simulink model "gm_sampleModel2003_1_sub"  (R2023a)
settings: Solver=VariableStepAuto  StartTime=0.0  StopTime=10.0  RelTol=1e-3
libraries: simulink x2, hdlsllib x1
settings Model: Creator=user1  LastModifiedBy=user1
settings OptimizationCC: BlockReduction=off  ConditionallyExecuteInputs=off
settings DebuggingCC: InheritedTsInSrcMsg=none

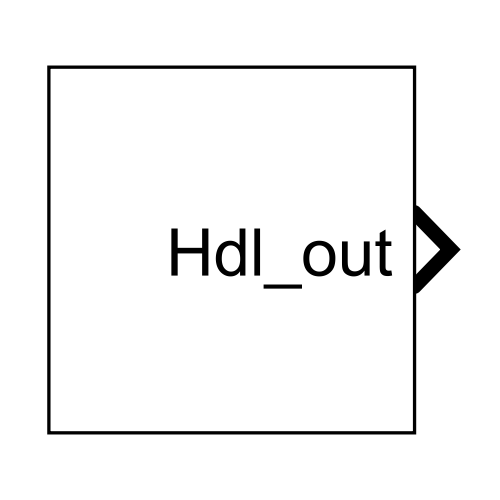
[thumbnail: Simulink's stored preview of the top-level diagram]
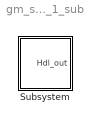
== system gm_sampleModel2003_1_sub ==
  Subsystem : Subsystem

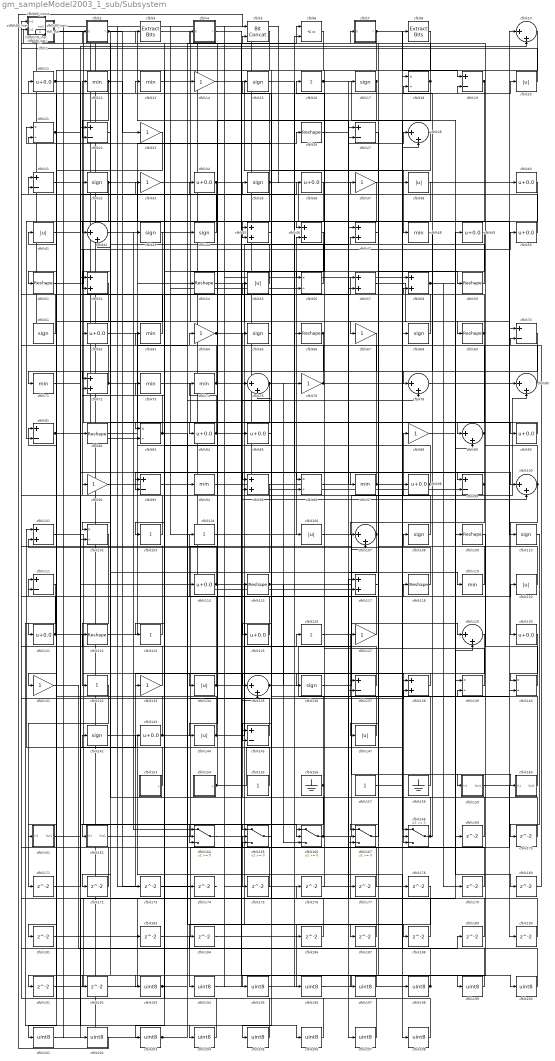
== system gm_sampleModel2003_1_sub/Subsystem ==
  cfblk1 : Subsystem  mask(Compare To Constant){relop=<=, const=double(3), OutDataTypeStr=uint8, ZeroCross=on}
      mask prompts: relop "Simulink:masks:Operator_MP"; const "Simulink:masks:ConstantValue_MP"; OutDataTypeStr "Simulink:masks:OutputDataType_MP"; ZeroCross "Simulink:masks:EnableZerocrossingDetection_MP"
      mask help: Simulink:masks:CompareToConstant_MD
      mask init:
      | OutDataTypeStr = 'uint8';
      | ZeroCross = 'on';
      | blkName = 'sampleModel2003_1_sub/Subsystem/cfblk1';
      | const = double(3);
      | const_str = '3.0';
      | const_val = double(3);
      | relop = '<=';
      | setValue = 'fixdt(0, 8)';
      | str = '<= 3';
      mask TypeOptions relop: == | ~= | < | <= | >= | >
      mask TypeOptions OutDataTypeStr: Simulink:masks:uint8 | Simulink:masks:boolean
      mask Callback ZeroCross: sl('zeroCrossEnable', gcbh);
      mask Display: disp(str)
  cfblk{10,28,42,75,78,80,89,100,107,129,135} (11 alike) : Sum  Inputs=|++  OutDataTypeStr=uint8
  cfblk{45..47,52,57..58,72,95,101,117,138} (11 alike) : Sum  OutDataTypeStr=uint8
  cfblk{18,21,56,83,96,102,139..140} (8 alike) : Product  Inputs=*/  OutDataTypeStr=uint8  RndMeth=Zero  SaturateOnIntegerOverflow=on
  cfblk{16,103..104,123,126,132} (6 alike) : Sum  Inputs=+  OutDataTypeStr=uint8
  cfblk{20,38,41,55,106,120,134,144,147} (9 alike) : Abs  OutDataTypeStr=uint8  SaturateOnIntegerOverflow=off
  cfblk{15,17,32,35,43..44,61,65,68,108,110,136,142} (13 alike) : Signum
  cfblk{26,51,54,59,66,69,82,109,115,118,122} (11 alike) : Reshape
  cfblk{11,34,36,40,49..50,62,84..85,90,98,114,121,125,130,143} (16 alike) : Bias  Bias=0.0  SaturateOnIntegerOverflow=off
  cfblk{19,22,27,31,70,81,93,99,111,137,145} (11 alike) : Sum  Inputs=+-  OutDataTypeStr=uint8
  cfblk113_inst : Subsystem
  cfblk116_inst : Subsystem
  cfblk{12..13,48,63,71,73..74,94,97,119} (10 alike) : MinMax  OutDataTypeStr=uint8
  cfblk124_inst : Subsystem
  cfblk{14,23,33,37,64,67,76,88,92,127,131,133} (12 alike) : Gain  OutDataTypeStr=uint8
  cfblk128_inst : Subsystem
  cfblk141_inst : Subsystem
  cfblk146_inst : Subsystem
  cfblk153 : Subsystem  mask(Counter Limited){uplimit=double(7), tsamp=double(-1)}
      mask prompts: uplimit "Simulink:masks:UpperLimit_MP"; tsamp "Simulink:masks:SampleTime_MP"
      mask help: Simulink:masks:CounterLimited_MD
      mask init:
      | nbits = double(8);
      | tsamp = double(-1);
      | uplimit = double(7);
  cfblk154 : Subsystem  mask(Counter Free-Running){NumBits=double(16), tsamp=double(-1)}
      mask prompts: NumBits "Simulink:masks:NumberOfBits_MP"; tsamp "Simulink:masks:SampleTime_MP"
      mask help: Simulink:masks:CounterFreeRunning_MD
  cfblk155 : Constant  OutDataTypeStr=uint8  SampleTime=-1
  cfblk156 : Ground
  cfblk157 : Constant  OutDataTypeStr=uint8  SampleTime=-1
  cfblk158 : Ground
  cfblk159 : Subsystem
  cfblk160 : Subsystem
  cfblk161 : Subsystem
  cfblk162 : Subsystem
  cfblk{164..168} (5 alike) : Switch  OutDataTypeStr=uint8  SaturateOnIntegerOverflow=off  InputSameDT=off
  cfblk{169..181,183..184,186..192} (22 alike) : Delay  SampleTime=1
  cfblk{193..208} (16 alike) : DataTypeConversion  OutDataTypeStr=uint8  SaturateOnIntegerOverflow=off  RndMeth=Floor
  cfblk2 : Subsystem  mask(Detect Rise Nonnegative){vinit=double(0), InputProcessing=Elements as channels (sample based), OutDataTypeStr=uint8}
      mask prompts: vinit "Simulink:masks:InitialCondition_MP"; InputProcessing "Simulink:masks:InputProcessing_MP"; OutDataTypeStr "Simulink:masks:OutputDataType_MP"
      mask help: Simulink:masks:DetectRiseNonnegative_MD
      mask init:
      | InputProcessing = 'Elements as channels (sample based)';
      | OutDataTypeStr = 'uint8';
      | vinit = double(0);
      mask TypeOptions InputProcessing: Simulink:masks:ColumnsAsChannelsFrameBased | Simulink:masks:ElementsAsChannelsSampleBased
      mask TypeOptions OutDataTypeStr: Simulink:masks:uint8 | Simulink:masks:boolean
      mask Display: fprintf('U >= 0\n&  NOT\nU/z >= 0')
  cfblk24_inst : Subsystem
  cfblk25_inst : Subsystem
  cfblk29_inst : Subsystem
  cfblk3 : simulink/Logic and Bit Operations/Extract Bits  bitsToExtract=Upper half  numBits=8  bitIdxRange=[0 7]  outScalingMode=Preserve fixed-point scaling
      settings: LibrarySourceBlock=|
      | hdlsllib/Logic and Bit
      | Operations/Extract Bits
  cfblk39_inst : Subsystem
  cfblk4 : Subsystem  mask(Detect Fall Nonpositive){vinit=double(0), InputProcessing=Elements as channels (sample based), OutDataTypeStr=uint8}
      mask prompts: vinit "Simulink:masks:InitialCondition_MP"; InputProcessing "Simulink:masks:InputProcessing_MP"; OutDataTypeStr "Simulink:masks:OutputDataType_MP"
      mask help: Simulink:masks:DetectFallNonpositive_MD
      mask init:
      | InputProcessing = 'Elements as channels (sample based)';
      | OutDataTypeStr = 'uint8';
      | vinit = double(0);
      mask TypeOptions InputProcessing: Simulink:masks:ColumnsAsChannelsFrameBased | Simulink:masks:ElementsAsChannelsSampleBased
      mask TypeOptions OutDataTypeStr: Simulink:masks:uint8 | Simulink:masks:boolean
      mask Display: fprintf('U <= 0\n&  NOT\nU/z <= 0')
  cfblk5 : hdlsllib/Logic and Bit Operations/Bit Concat  numInputs=2
  cfblk6 : RelationalOperator  Operator=<=  OutDataTypeStr=boolean  InputSameDT=off
  cfblk60_inst : Subsystem
  cfblk7 : Subsystem  mask(Detect Rise Positive){vinit=double(0), InputProcessing=Elements as channels (sample based), OutDataTypeStr=uint8}
      mask prompts: vinit "Simulink:masks:InitialCondition_MP"; InputProcessing "Simulink:masks:InputProcessing_MP"; OutDataTypeStr "Simulink:masks:OutputDataType_MP"
      mask help: Simulink:masks:DetectRisePositive_MD
      mask init:
      | InputProcessing = 'Elements as channels (sample based)';
      | OutDataTypeStr = 'uint8';
      | vinit = double(0);
      mask TypeOptions InputProcessing: Simulink:masks:ColumnsAsChannelsFrameBased | Simulink:masks:ElementsAsChannelsSampleBased
      mask TypeOptions OutDataTypeStr: Simulink:masks:uint8 | Simulink:masks:boolean
      mask Display: fprintf('U > 0\n&  NOT\nU/z > 0')
  cfblk79_inst : Subsystem
  cfblk8 : simulink/Logic and Bit Operations/Extract Bits  bitsToExtract=Upper half  numBits=8  bitIdxRange=[0 7]  outScalingMode=Preserve fixed-point scaling
      settings: LibrarySourceBlock=|
      | hdlsllib/Logic and Bit
      | Operations/Extract Bits
  cfblk86_inst : Subsystem
  cfblk9_inst : Subsystem
  Hdl_out : Outport  OutDataTypeStr=uint8  SampleTime=1
  wires:
  cfblk1/1(y) -> cfblk89/1, cfblk45/2
  cfblk10/1 -> cfblk75/2
  cfblk100/1 -> cfblk47/2, cfblk130/1, cfblk128_inst/2(in2)
  cfblk101/1 -> cfblk166/2
  cfblk102/1 -> cfblk132/1
  cfblk103/1 -> cfblk12/1
  cfblk104/1 -> cfblk46/2
  cfblk106/1 -> cfblk129/1
  cfblk107/1 -> cfblk25_inst/2(in2), cfblk172/1
  cfblk108/1 -> cfblk35/1
  cfblk109/1 -> cfblk191/1
  cfblk11/1 -> cfblk164/3, cfblk97/1
  cfblk110/1 -> cfblk170/1
  cfblk111/1 -> cfblk204/1
  cfblk113_inst/1(out1) -> cfblk40/1
  cfblk114/1 -> cfblk29_inst/2(in2), cfblk188/1
  cfblk115/1 -> cfblk80/2, cfblk166/3, cfblk159/1(In1)
  cfblk116_inst/1(out1) -> cfblk94/1
  cfblk117/1 -> cfblk7/1(U)
  cfblk118/1 -> cfblk101/2
  cfblk119/1 -> cfblk29_inst/1(in1)
  cfblk12/1 -> cfblk22/2, cfblk23/1
  cfblk120/1 -> cfblk92/1
  cfblk121/1 -> cfblk60_inst/1(in1), cfblk168/3
  cfblk122/1 -> cfblk26/1
  cfblk123/1 -> cfblk41/1
  cfblk124_inst/1(out1) -> cfblk178/1
  cfblk125/1 -> cfblk141_inst/1(in1)
  cfblk126/1 -> cfblk49/1
  cfblk127/1 -> cfblk104/1
  cfblk128_inst/1(out1) -> cfblk43/1
  cfblk129/1 -> cfblk173/1
  cfblk13/1 -> cfblk67/1
  cfblk130/1 -> cfblk140/1
  cfblk131/1 -> cfblk189/1
  cfblk132/1 -> cfblk171/1
  cfblk133/1 -> cfblk39_inst/2(in2)
  cfblk134/1 -> cfblk21/2, cfblk126/1
  cfblk135/1 -> cfblk107/2, cfblk76/1, cfblk139/2
  cfblk136/1 -> cfblk88/1
  cfblk137/1 -> cfblk146_inst/2(in2)
  cfblk138/1 -> cfblk136/1
  cfblk139/1 -> cfblk16/1
  cfblk14/1 -> cfblk48/1
  cfblk140/1 -> cfblk9_inst/1(in1)
  cfblk141_inst/1(out1) -> cfblk82/1
  cfblk142/1 -> cfblk208/1
  cfblk143/1 -> cfblk68/1, cfblk42/2
  cfblk144/1 -> cfblk31/1, cfblk27/1, cfblk122/1
  cfblk145/1 -> cfblk9_inst/2(in2)
  cfblk146_inst/1(out1) -> cfblk202/1
  cfblk147/1 -> cfblk127/1
  cfblk15/1 -> cfblk90/1
  cfblk153/1(y) -> cfblk142/1
  cfblk154/1(y) -> cfblk8/1, cfblk64/1
  cfblk155/1 -> cfblk101/1
  cfblk156/1 -> cfblk21/1, cfblk162/1(In1)
  cfblk157/1 -> cfblk28/2
  cfblk158/1 -> cfblk137/1
  cfblk159/1(Out1) -> cfblk190/1
  cfblk16/1 -> cfblk168/1, cfblk109/1
  cfblk160/1(Out1) -> cfblk32/1
  cfblk161/1(Out1) -> cfblk143/1
  cfblk162/1(Out1) -> cfblk138/2
  cfblk164/1 -> cfblk175/1
  cfblk165/1 -> cfblk195/1
  cfblk166/1 -> cfblk70/1, cfblk2/1(U)
  cfblk167/1 -> cfblk37/1
  cfblk168/1 -> cfblk65/1, cfblk108/1
  cfblk169/1 -> cfblk18/2
  cfblk17/1 -> cfblk84/1, cfblk135/1
  cfblk170/1 -> cfblk95/2
  cfblk171/1 -> cfblk10/2
  cfblk172/1 -> cfblk24_inst/2(in2)
  cfblk173/1 -> cfblk89/2
  cfblk174/1 -> cfblk1/1(u)
  cfblk175/1 -> cfblk39_inst/1(in1)
  cfblk176/1 -> cfblk96/2
  cfblk177/1 -> cfblk75/1
  cfblk178/1 -> cfblk194/1
  cfblk179/1 -> cfblk141_inst/2(in2)
  cfblk18/1 -> cfblk27/2, cfblk145/2, cfblk116_inst/1(in1)
  cfblk180/1 -> cfblk70/2
  cfblk181/1 -> cfblk117/1
  cfblk183/1 -> cfblk140/2
  cfblk184/1 -> cfblk196/1
  cfblk186/1 -> cfblk165/3
  cfblk187/1 -> cfblk81/1
  cfblk188/1 -> cfblk167/2
  cfblk189/1 -> cfblk168/2
  cfblk19/1 -> cfblk81/2, cfblk107/1
  cfblk190/1 -> cfblk116_inst/2(in2)
  cfblk191/1 -> cfblk139/1
  cfblk192/1 -> cfblk165/2
  cfblk193/1 -> cfblk78/2, cfblk57/1, cfblk120/1, cfblk118/1
  cfblk194/1 -> cfblk6/1
  cfblk195/1 -> cfblk6/2
  cfblk196/1 -> cfblk200/1
  cfblk197/1 -> cfblk184/1
  cfblk198/1 -> cfblk86_inst/2(in2), cfblk18/1
  cfblk199/1 -> cfblk79_inst/1(in1)
  cfblk2/1(Y) -> cfblk42/1, cfblk137/2
  cfblk20/1 -> cfblk146_inst/1(in1)
  cfblk200/1 -> cfblk79_inst/2(in2)
  cfblk201/1 -> cfblk176/1
  cfblk202/1 -> cfblk5/1
  cfblk203/1 -> cfblk5/2, Hdl_out/1
  cfblk204/1 -> cfblk124_inst/1(in1)
  cfblk205/1 -> cfblk111/1
  cfblk206/1 -> cfblk111/2
  cfblk207/1 -> cfblk124_inst/2(in2)
  cfblk208/1 -> cfblk3/1
  cfblk21/1 -> cfblk46/1, cfblk206/1, cfblk183/1
  cfblk22/1 -> cfblk102/1
  cfblk23/1 -> cfblk181/1
  cfblk24_inst/1(out1) -> cfblk117/2, cfblk83/2
  cfblk25_inst/1(out1) -> cfblk106/1
  cfblk26/1 -> cfblk119/1
  cfblk27/1 -> cfblk187/1
  cfblk28/1 -> cfblk45/1
  cfblk29_inst/1(out1) -> cfblk58/1
  cfblk3/1 -> cfblk207/1
  cfblk31/1 -> cfblk114/1
  cfblk32/1 -> cfblk177/1, cfblk102/2
  cfblk33/1 -> cfblk59/1
  cfblk34/1 -> cfblk203/1, cfblk138/1
  cfblk35/1 -> cfblk80/1, cfblk144/1, cfblk113_inst/1(in1)
  cfblk36/1 -> cfblk52/2
  cfblk37/1 -> cfblk51/1
  cfblk38/1 -> cfblk134/1
  cfblk39_inst/1(out1) -> cfblk44/1, cfblk56/2
  cfblk4/1(Y) -> cfblk199/1
  cfblk40/1 -> cfblk161/1(In1)
  cfblk41/1 -> cfblk69/1
  cfblk42/1 -> cfblk164/1
  cfblk43/1 -> cfblk131/1
  cfblk44/1 -> cfblk24_inst/1(in1)
  cfblk45/1 -> cfblk165/1
  cfblk46/1 -> cfblk123/1
  cfblk47/1 -> cfblk147/1
  cfblk48/1 -> cfblk78/1
  cfblk49/1 -> cfblk197/1
  cfblk5/1 -> cfblk201/1
  cfblk50/1 -> cfblk11/1
  cfblk51/1 -> cfblk17/1
  cfblk52/1 -> cfblk121/1
  cfblk54/1 -> cfblk110/1
  cfblk55/1 -> cfblk25_inst/1(in1)
  cfblk56/1 -> cfblk13/1
  cfblk57/1 -> cfblk169/1
  cfblk58/1 -> cfblk180/1, cfblk179/1
  cfblk59/1 -> cfblk4/1(U)
  cfblk6/1 -> cfblk193/1
  cfblk60_inst/1(out1) -> cfblk174/1
  cfblk61/1 -> cfblk86_inst/1(in1)
  cfblk62/1 -> cfblk115/1
  cfblk63/1 -> cfblk52/1
  cfblk64/1 -> cfblk20/1, cfblk100/1
  cfblk65/1 -> cfblk15/1
  cfblk66/1 -> cfblk95/1, cfblk93/2
  cfblk67/1 -> cfblk72/1
  cfblk68/1 -> cfblk60_inst/2(in2)
  cfblk69/1 -> cfblk58/2, cfblk205/1, cfblk103/1
  cfblk7/1(Y) -> cfblk19/1, cfblk56/1
  cfblk70/1 -> cfblk71/1
  cfblk71/1 -> cfblk50/1
  cfblk72/1 -> cfblk54/1, cfblk22/1
  cfblk73/1 -> cfblk129/2
  cfblk74/1 -> cfblk62/1, cfblk135/2
  cfblk75/1 -> cfblk99/1, cfblk192/1
  cfblk76/1 -> cfblk57/2, cfblk31/2, cfblk19/2, cfblk63/1
  cfblk78/1 -> cfblk10/1
  cfblk79_inst/1(out1) -> cfblk198/1
  cfblk8/1 -> cfblk145/1
  cfblk80/1 -> cfblk128_inst/1(in1)
  cfblk81/1 -> cfblk55/1, cfblk36/1
  cfblk82/1 -> cfblk14/1
  cfblk83/1 -> cfblk72/2, cfblk166/1, cfblk186/1
  cfblk84/1 -> cfblk66/1, cfblk74/1
  cfblk85/1 -> cfblk125/1
  cfblk86_inst/1(out1) -> cfblk98/1
  cfblk88/1 -> cfblk160/1(In1)
  cfblk89/1 -> cfblk167/3, cfblk33/1
  cfblk9_inst/1(out1) -> cfblk99/2, cfblk61/1
  cfblk90/1 -> cfblk83/1
  cfblk92/1 -> cfblk85/1
  cfblk93/1 -> cfblk164/2
  cfblk94/1 -> cfblk100/2
  cfblk95/1 -> cfblk133/1
  cfblk96/1 -> cfblk28/1
  cfblk97/1 -> cfblk38/1, cfblk34/1, cfblk113_inst/2(in2)
  cfblk98/1 -> cfblk47/1, cfblk96/1, cfblk73/1
  cfblk99/1 -> cfblk93/1, cfblk167/1

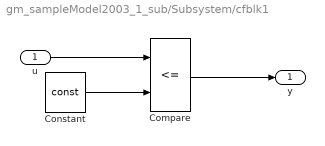
== system gm_sampleModel2003_1_sub/Subsystem/cfblk1 ==
  u : Inport  OutDataTypeStr=uint8  SampleTime=1
  Compare : RelationalOperator  Operator=<=  OutDataTypeStr=fixdt(0, 8)
  Constant : Constant  DisableCoverage=on  Value=const  OutDataTypeStr=Inherit: Inherit via back propagation  SampleTime=-1
  y : Outport  SampleTime=1
  wires:
  u/1 -> Compare/1
  Compare/1 -> y/1
  Constant/1 -> Compare/2

== system gm_sampleModel2003_1_sub/Subsystem/cfblk113_inst ==
  in1 : Inport  OutDataTypeStr=uint8  SampleTime=1
  in2 : Inport  Port=2  OutDataTypeStr=uint8  SampleTime=1
  mul_cfblk113_dotp_mulcomp : Product  Inputs=**  OutDataTypeStr=uint8  SampleTime=1
  out1 : Outport  OutDataTypeStr=uint8  SampleTime=1
  wires:
  in1/1 -> mul_cfblk113_dotp_mulcomp/1
  in2/1 -> mul_cfblk113_dotp_mulcomp/2
  mul_cfblk113_dotp_mulcomp/1 -> out1/1

== system gm_sampleModel2003_1_sub/Subsystem/cfblk116_inst ==
  in1 : Inport  OutDataTypeStr=uint8  SampleTime=1
  in2 : Inport  Port=2  OutDataTypeStr=uint8  SampleTime=1
  mul_cfblk116_dotp_mulcomp : Product  Inputs=**  OutDataTypeStr=uint8  SampleTime=1
  out1 : Outport  OutDataTypeStr=uint8  SampleTime=1
  wires:
  in1/1 -> mul_cfblk116_dotp_mulcomp/1
  in2/1 -> mul_cfblk116_dotp_mulcomp/2
  mul_cfblk116_dotp_mulcomp/1 -> out1/1

== system gm_sampleModel2003_1_sub/Subsystem/cfblk124_inst ==
  in1 : Inport  OutDataTypeStr=uint8  SampleTime=1
  in2 : Inport  Port=2  OutDataTypeStr=uint8  SampleTime=1
  mul_cfblk124_dotp_mulcomp : Product  Inputs=**  OutDataTypeStr=uint8  SampleTime=1
  out1 : Outport  OutDataTypeStr=uint8  SampleTime=1
  wires:
  in1/1 -> mul_cfblk124_dotp_mulcomp/1
  in2/1 -> mul_cfblk124_dotp_mulcomp/2
  mul_cfblk124_dotp_mulcomp/1 -> out1/1

== system gm_sampleModel2003_1_sub/Subsystem/cfblk128_inst ==
  in1 : Inport  OutDataTypeStr=uint8  SampleTime=1
  in2 : Inport  Port=2  OutDataTypeStr=uint8  SampleTime=1
  mul_cfblk128_dotp_mulcomp : Product  Inputs=**  OutDataTypeStr=uint8  SampleTime=1
  out1 : Outport  OutDataTypeStr=uint8  SampleTime=1
  wires:
  in1/1 -> mul_cfblk128_dotp_mulcomp/1
  in2/1 -> mul_cfblk128_dotp_mulcomp/2
  mul_cfblk128_dotp_mulcomp/1 -> out1/1

== system gm_sampleModel2003_1_sub/Subsystem/cfblk141_inst ==
  in1 : Inport  OutDataTypeStr=uint8  SampleTime=1
  in2 : Inport  Port=2  OutDataTypeStr=uint8  SampleTime=1
  mul_cfblk141_dotp_mulcomp : Product  Inputs=**  OutDataTypeStr=uint8  SampleTime=1
  out1 : Outport  OutDataTypeStr=uint8  SampleTime=1
  wires:
  in1/1 -> mul_cfblk141_dotp_mulcomp/1
  in2/1 -> mul_cfblk141_dotp_mulcomp/2
  mul_cfblk141_dotp_mulcomp/1 -> out1/1

== system gm_sampleModel2003_1_sub/Subsystem/cfblk146_inst ==
  in1 : Inport  OutDataTypeStr=uint8  SampleTime=1
  in2 : Inport  Port=2  OutDataTypeStr=uint8  SampleTime=1
  mul_cfblk146_dotp_mulcomp : Product  Inputs=**  OutDataTypeStr=uint8  SampleTime=1
  out1 : Outport  OutDataTypeStr=uint8  SampleTime=1
  wires:
  in1/1 -> mul_cfblk146_dotp_mulcomp/1
  in2/1 -> mul_cfblk146_dotp_mulcomp/2
  mul_cfblk146_dotp_mulcomp/1 -> out1/1

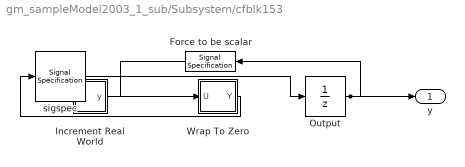
== system gm_sampleModel2003_1_sub/Subsystem/cfblk153 ==
  Force to be scalar : SignalSpecification  DisableCoverage=on  Dimensions=1
  Increment Real World : Subsystem  mask(Real World Value Increment){}
      mask help: Simulink:masks:RealWorldValueIncrement_MD
      mask Display: disp('V++')
  Output : UnitDelay  InitialCondition=0.0  SampleTime=tsamp  HasFrameUpgradeWarning=on
  Wrap To Zero : Subsystem  mask(Wrap To Zero){Threshold=double(7)}
      mask prompts: Threshold "Simulink:masks:Threshold_MP"
      mask help: Simulink:masks:WrapToZero_MD
  sigspec : SignalSpecification  OutDataTypeStr=uint8  Dimensions=1
  y : Outport  SampleTime=1
  wires:
  Force to be scalar/1 -> Increment Real World/1(u)
  Increment Real World/1(y) -> Wrap To Zero/1(U)
  Output/1 -> Force to be scalar/1, y/1
  Wrap To Zero/1(Y) -> sigspec/1
  sigspec/1 -> Output/1

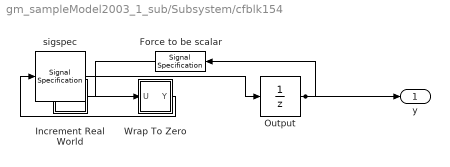
== system gm_sampleModel2003_1_sub/Subsystem/cfblk154 ==
  Force to be scalar : SignalSpecification  DisableCoverage=on  Dimensions=1
  Increment Real World : Subsystem  mask(Real World Value Increment){}
      mask help: Simulink:masks:RealWorldValueIncrement_MD
      mask Display: disp('V++')
  Output : UnitDelay  InitialCondition=0.0  SampleTime=tsamp  HasFrameUpgradeWarning=on
  Wrap To Zero : Subsystem  mask(Wrap To Zero){Threshold=double(65535)}
      mask prompts: Threshold "Simulink:masks:Threshold_MP"
      mask help: Simulink:masks:WrapToZero_MD
  sigspec : SignalSpecification  OutDataTypeStr=uint16  Dimensions=1
  y : Outport  SampleTime=1
  wires:
  Force to be scalar/1 -> Increment Real World/1(u)
  Increment Real World/1(y) -> Wrap To Zero/1(U)
  Output/1 -> Force to be scalar/1, y/1
  Wrap To Zero/1(Y) -> sigspec/1
  sigspec/1 -> Output/1

== system gm_sampleModel2003_1_sub/Subsystem/cfblk159 ==
  In1 : Inport  OutDataTypeStr=uint8  PortDimensions=1  SampleTime=1
  Out1 : Outport  SampleTime=1
  wires:
  In1/1 -> Out1/1

== system gm_sampleModel2003_1_sub/Subsystem/cfblk160 ==
  In1 : Inport  OutDataTypeStr=uint8  PortDimensions=1  SampleTime=1
  Out1 : Outport  SampleTime=1
  wires:
  In1/1 -> Out1/1

== system gm_sampleModel2003_1_sub/Subsystem/cfblk161 ==
  In1 : Inport  OutDataTypeStr=uint8  PortDimensions=1  SampleTime=1
  Out1 : Outport  SampleTime=1
  wires:
  In1/1 -> Out1/1

== system gm_sampleModel2003_1_sub/Subsystem/cfblk162 ==
  In1 : Inport  OutDataTypeStr=uint8  PortDimensions=1  SampleTime=1
  Out1 : Outport  SampleTime=1
  wires:
  In1/1 -> Out1/1

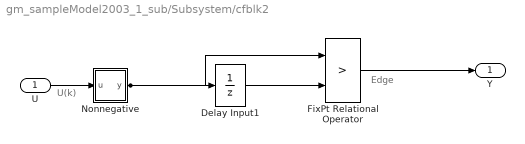
== system gm_sampleModel2003_1_sub/Subsystem/cfblk2 ==
  note: U(k)
  note: Edge
  U : Inport  OutDataTypeStr=uint8  SampleTime=1
  Delay Input1 : UnitDelay  Description=Store in Global RAM  DisableCoverage=on  InitialCondition=vinit  SampleTime=-1  HasFrameUpgradeWarning=on
  FixPt Relational Operator : RelationalOperator  Operator=>  OutDataTypeStr=fixdt(0, 8)  ZeroCross=off  InputSameDT=off
  Nonnegative : Subsystem  mask(Compare To Zero){relop=>=, OutDataTypeStr=boolean, ZeroCross=off}
      mask prompts: relop "Simulink:masks:Operator_MP"; OutDataTypeStr "Simulink:masks:OutputDataType_MP"; ZeroCross "Simulink:masks:EnableZerocrossingDetection_MP"
      mask help: Simulink:masks:CompareToZero_MD
      mask init:
      | OutDataTypeStr = 'boolean';
      | ZeroCross = 'off';
      | blkName = 'sampleModel2003_1_sub/Subsystem/cfblk2/Nonnegative';
      | relop = '>=';
      | setValue = 'boolean';
      mask TypeOptions relop: == | ~= | < | <= | >= | >
      mask TypeOptions OutDataTypeStr: Simulink:masks:uint8 | Simulink:masks:boolean
      mask Callback ZeroCross: sl('zeroCrossEnable', gcbh);
      mask Display: disp([relop,' 0'])
  Y : Outport  SampleTime=1
  wires:
  U/1 -> Nonnegative/1(u)
  Delay Input1/1 -> FixPt Relational Operator/2
  FixPt Relational Operator/1 -> Y/1
  Nonnegative/1(y) -> FixPt Relational Operator/1, Delay Input1/1

== system gm_sampleModel2003_1_sub/Subsystem/cfblk24_inst ==
  in1 : Inport  OutDataTypeStr=uint8  SampleTime=1
  in2 : Inport  Port=2  OutDataTypeStr=uint8  SampleTime=1
  mul_cfblk24_dotp_mulcomp : Product  Inputs=**  OutDataTypeStr=uint8  SampleTime=1
  out1 : Outport  OutDataTypeStr=uint8  SampleTime=1
  wires:
  in1/1 -> mul_cfblk24_dotp_mulcomp/1
  in2/1 -> mul_cfblk24_dotp_mulcomp/2
  mul_cfblk24_dotp_mulcomp/1 -> out1/1

== system gm_sampleModel2003_1_sub/Subsystem/cfblk25_inst ==
  in1 : Inport  OutDataTypeStr=uint8  SampleTime=1
  in2 : Inport  Port=2  OutDataTypeStr=uint8  SampleTime=1
  mul_cfblk25_dotp_mulcomp : Product  Inputs=**  OutDataTypeStr=uint8  SampleTime=1
  out1 : Outport  OutDataTypeStr=uint8  SampleTime=1
  wires:
  in1/1 -> mul_cfblk25_dotp_mulcomp/1
  in2/1 -> mul_cfblk25_dotp_mulcomp/2
  mul_cfblk25_dotp_mulcomp/1 -> out1/1

== system gm_sampleModel2003_1_sub/Subsystem/cfblk29_inst ==
  in1 : Inport  OutDataTypeStr=uint8  SampleTime=1
  in2 : Inport  Port=2  OutDataTypeStr=uint8  SampleTime=1
  mul_cfblk29_dotp_mulcomp : Product  Inputs=**  OutDataTypeStr=uint8  SampleTime=1
  out1 : Outport  OutDataTypeStr=uint8  SampleTime=1
  wires:
  in1/1 -> mul_cfblk29_dotp_mulcomp/1
  in2/1 -> mul_cfblk29_dotp_mulcomp/2
  mul_cfblk29_dotp_mulcomp/1 -> out1/1

== system gm_sampleModel2003_1_sub/Subsystem/cfblk39_inst ==
  in1 : Inport  OutDataTypeStr=uint8  SampleTime=1
  in2 : Inport  Port=2  OutDataTypeStr=uint8  SampleTime=1
  mul_cfblk39_dotp_mulcomp : Product  Inputs=**  OutDataTypeStr=uint8  SampleTime=1
  out1 : Outport  OutDataTypeStr=uint8  SampleTime=1
  wires:
  in1/1 -> mul_cfblk39_dotp_mulcomp/1
  in2/1 -> mul_cfblk39_dotp_mulcomp/2
  mul_cfblk39_dotp_mulcomp/1 -> out1/1

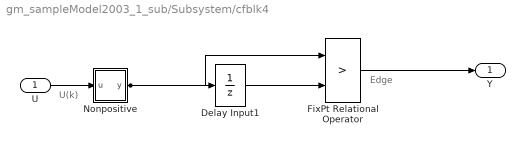
== system gm_sampleModel2003_1_sub/Subsystem/cfblk4 ==
  note: U(k)
  note: Edge
  U : Inport  OutDataTypeStr=uint8  SampleTime=1
  Delay Input1 : UnitDelay  Description=Store in Global RAM  DisableCoverage=on  InitialCondition=vinit  SampleTime=-1  HasFrameUpgradeWarning=on
  FixPt Relational Operator : RelationalOperator  Operator=>  OutDataTypeStr=fixdt(0, 8)  ZeroCross=off  InputSameDT=off
  Nonpositive : Subsystem  mask(Compare To Zero){relop=<=, OutDataTypeStr=boolean, ZeroCross=off}
      mask prompts: relop "Simulink:masks:Operator_MP"; OutDataTypeStr "Simulink:masks:OutputDataType_MP"; ZeroCross "Simulink:masks:EnableZerocrossingDetection_MP"
      mask help: Simulink:masks:CompareToZero_MD
      mask init:
      | OutDataTypeStr = 'boolean';
      | ZeroCross = 'off';
      | blkName = 'sampleModel2003_1_sub/Subsystem/cfblk4/Nonpositive';
      | relop = '<=';
      | setValue = 'boolean';
      mask TypeOptions relop: == | ~= | < | <= | >= | >
      mask TypeOptions OutDataTypeStr: Simulink:masks:uint8 | Simulink:masks:boolean
      mask Callback ZeroCross: sl('zeroCrossEnable', gcbh);
      mask Display: disp([relop,' 0'])
  Y : Outport  SampleTime=1
  wires:
  U/1 -> Nonpositive/1(u)
  Delay Input1/1 -> FixPt Relational Operator/2
  FixPt Relational Operator/1 -> Y/1
  Nonpositive/1(y) -> FixPt Relational Operator/1, Delay Input1/1

== system gm_sampleModel2003_1_sub/Subsystem/cfblk60_inst ==
  in1 : Inport  OutDataTypeStr=uint8  SampleTime=1
  in2 : Inport  Port=2  OutDataTypeStr=uint8  SampleTime=1
  mul_cfblk60_dotp_mulcomp : Product  Inputs=**  OutDataTypeStr=uint8  SampleTime=1
  out1 : Outport  OutDataTypeStr=uint8  SampleTime=1
  wires:
  in1/1 -> mul_cfblk60_dotp_mulcomp/1
  in2/1 -> mul_cfblk60_dotp_mulcomp/2
  mul_cfblk60_dotp_mulcomp/1 -> out1/1

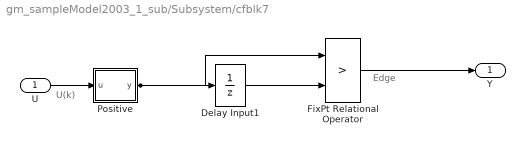
== system gm_sampleModel2003_1_sub/Subsystem/cfblk7 ==
  note: U(k)
  note: Edge
  U : Inport  OutDataTypeStr=uint8  SampleTime=1
  Delay Input1 : UnitDelay  Description=Store in Global RAM  DisableCoverage=on  InitialCondition=vinit  SampleTime=-1  HasFrameUpgradeWarning=on
  FixPt Relational Operator : RelationalOperator  Operator=>  OutDataTypeStr=fixdt(0, 8)  ZeroCross=off  InputSameDT=off
  Positive : Subsystem  mask(Compare To Zero){relop=>, OutDataTypeStr=boolean, ZeroCross=off}
      mask prompts: relop "Simulink:masks:Operator_MP"; OutDataTypeStr "Simulink:masks:OutputDataType_MP"; ZeroCross "Simulink:masks:EnableZerocrossingDetection_MP"
      mask help: Simulink:masks:CompareToZero_MD
      mask init:
      | OutDataTypeStr = 'boolean';
      | ZeroCross = 'off';
      | blkName = 'sampleModel2003_1_sub/Subsystem/cfblk7/Positive';
      | relop = '>';
      | setValue = 'boolean';
      mask TypeOptions relop: == | ~= | < | <= | >= | >
      mask TypeOptions OutDataTypeStr: Simulink:masks:uint8 | Simulink:masks:boolean
      mask Callback ZeroCross: sl('zeroCrossEnable', gcbh);
      mask Display: disp([relop,' 0'])
  Y : Outport  SampleTime=1
  wires:
  U/1 -> Positive/1(u)
  Delay Input1/1 -> FixPt Relational Operator/2
  FixPt Relational Operator/1 -> Y/1
  Positive/1(y) -> FixPt Relational Operator/1, Delay Input1/1

== system gm_sampleModel2003_1_sub/Subsystem/cfblk79_inst ==
  in1 : Inport  OutDataTypeStr=uint8  SampleTime=1
  in2 : Inport  Port=2  OutDataTypeStr=uint8  SampleTime=1
  mul_cfblk79_dotp_mulcomp : Product  Inputs=**  OutDataTypeStr=uint8  SampleTime=1
  out1 : Outport  OutDataTypeStr=uint8  SampleTime=1
  wires:
  in1/1 -> mul_cfblk79_dotp_mulcomp/1
  in2/1 -> mul_cfblk79_dotp_mulcomp/2
  mul_cfblk79_dotp_mulcomp/1 -> out1/1

== system gm_sampleModel2003_1_sub/Subsystem/cfblk86_inst ==
  in1 : Inport  OutDataTypeStr=uint8  SampleTime=1
  in2 : Inport  Port=2  OutDataTypeStr=uint8  SampleTime=1
  mul_cfblk86_dotp_mulcomp : Product  Inputs=**  OutDataTypeStr=uint8  SampleTime=1
  out1 : Outport  OutDataTypeStr=uint8  SampleTime=1
  wires:
  in1/1 -> mul_cfblk86_dotp_mulcomp/1
  in2/1 -> mul_cfblk86_dotp_mulcomp/2
  mul_cfblk86_dotp_mulcomp/1 -> out1/1

== system gm_sampleModel2003_1_sub/Subsystem/cfblk9_inst ==
  in1 : Inport  OutDataTypeStr=uint8  SampleTime=1
  in2 : Inport  Port=2  OutDataTypeStr=uint8  SampleTime=1
  mul_cfblk9_dotp_mulcomp : Product  Inputs=**  OutDataTypeStr=uint8  SampleTime=1
  out1 : Outport  OutDataTypeStr=uint8  SampleTime=1
  wires:
  in1/1 -> mul_cfblk9_dotp_mulcomp/1
  in2/1 -> mul_cfblk9_dotp_mulcomp/2
  mul_cfblk9_dotp_mulcomp/1 -> out1/1

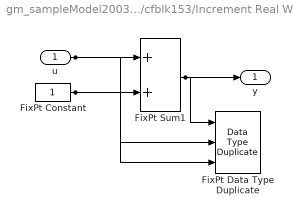
== system gm_sampleModel2003_1_sub/Subsystem/cfblk153/Increment Real World ==
  u : Inport  OutDataTypeStr=uint8  SampleTime=1
  FixPt Constant : Constant  DisableCoverage=on  OutDataTypeStr=Inherit: Inherit via back propagation  SampleTime=-1
  FixPt Data Type Duplicate : DataTypeDuplicate  DisableCoverage=on  NumInputPorts=3
  FixPt Sum1 : Sum  InputSameDT=on  OutDataTypeStr=Inherit: Inherit via back propagation  LockScale=on
  y : Outport  SampleTime=1
  wires:
  u/1 -> FixPt Sum1/1, FixPt Data Type Duplicate/2
  FixPt Constant/1 -> FixPt Sum1/2, FixPt Data Type Duplicate/3
  FixPt Sum1/1 -> FixPt Data Type Duplicate/1, y/1

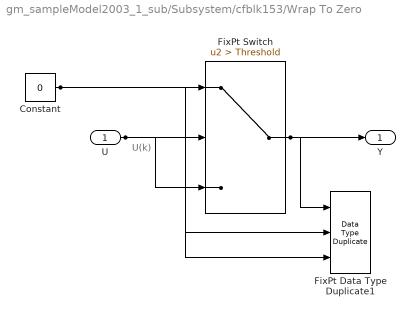
== system gm_sampleModel2003_1_sub/Subsystem/cfblk153/Wrap To Zero ==
  note: U(k)
  U : Inport  OutDataTypeStr=uint8  SampleTime=1
  Constant : Constant  DisableCoverage=on  Value=0  OutDataTypeStr=Inherit: Inherit via back propagation  SampleTime=-1
  FixPt Data Type Duplicate1 : DataTypeDuplicate  DisableCoverage=on  NumInputPorts=3
  FixPt Switch : Switch  Criteria=u2 > Threshold  Threshold=Threshold  OutDataTypeStr=Inherit: Inherit via back propagation  ZeroCross=off  SaturateOnIntegerOverflow=off  InputSameDT=off
  Y : Outport  SampleTime=1
  wires:
  U/1 -> FixPt Switch/3, FixPt Switch/2, FixPt Data Type Duplicate1/2
  Constant/1 -> FixPt Switch/1, FixPt Data Type Duplicate1/3
  FixPt Switch/1 -> FixPt Data Type Duplicate1/1, Y/1

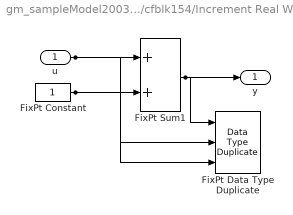
== system gm_sampleModel2003_1_sub/Subsystem/cfblk154/Increment Real World ==
  u : Inport  OutDataTypeStr=uint16  SampleTime=1
  FixPt Constant : Constant  DisableCoverage=on  OutDataTypeStr=Inherit: Inherit via back propagation  SampleTime=-1
  FixPt Data Type Duplicate : DataTypeDuplicate  DisableCoverage=on  NumInputPorts=3
  FixPt Sum1 : Sum  InputSameDT=on  OutDataTypeStr=Inherit: Inherit via back propagation  LockScale=on
  y : Outport  SampleTime=1
  wires:
  u/1 -> FixPt Sum1/1, FixPt Data Type Duplicate/2
  FixPt Constant/1 -> FixPt Sum1/2, FixPt Data Type Duplicate/3
  FixPt Sum1/1 -> FixPt Data Type Duplicate/1, y/1

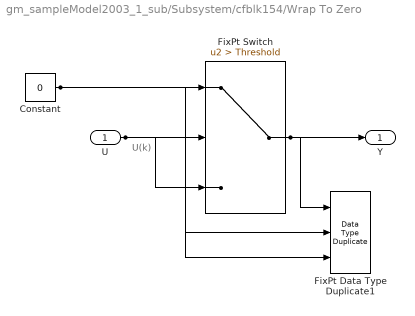
== system gm_sampleModel2003_1_sub/Subsystem/cfblk154/Wrap To Zero ==
  note: U(k)
  U : Inport  OutDataTypeStr=uint16  SampleTime=1
  Constant : Constant  DisableCoverage=on  Value=0  OutDataTypeStr=Inherit: Inherit via back propagation  SampleTime=-1
  FixPt Data Type Duplicate1 : DataTypeDuplicate  DisableCoverage=on  NumInputPorts=3
  FixPt Switch : Switch  Criteria=u2 > Threshold  Threshold=Threshold  OutDataTypeStr=Inherit: Inherit via back propagation  ZeroCross=off  SaturateOnIntegerOverflow=off  InputSameDT=off
  Y : Outport  SampleTime=1
  wires:
  U/1 -> FixPt Switch/3, FixPt Switch/2, FixPt Data Type Duplicate1/2
  Constant/1 -> FixPt Switch/1, FixPt Data Type Duplicate1/3
  FixPt Switch/1 -> FixPt Data Type Duplicate1/1, Y/1

== system gm_sampleModel2003_1_sub/Subsystem/cfblk2/Nonnegative ==
  u : Inport  OutDataTypeStr=uint8  SampleTime=1
  Compare : RelationalOperator  OutDataTypeStr=boolean  ZeroCross=off
  Constant : Constant  DisableCoverage=on  Value=0  OutDataTypeStr=Inherit: Inherit via back propagation  SampleTime=-1  PreserveConstantTs=on
  y : Outport  SampleTime=1
  wires:
  u/1 -> Compare/1
  Compare/1 -> y/1
  Constant/1 -> Compare/2

== system gm_sampleModel2003_1_sub/Subsystem/cfblk4/Nonpositive ==
  u : Inport  OutDataTypeStr=uint8  SampleTime=1
  Compare : RelationalOperator  Operator=<=  OutDataTypeStr=boolean  ZeroCross=off
  Constant : Constant  DisableCoverage=on  Value=0  OutDataTypeStr=Inherit: Inherit via back propagation  SampleTime=-1  PreserveConstantTs=on
  y : Outport  SampleTime=1
  wires:
  u/1 -> Compare/1
  Compare/1 -> y/1
  Constant/1 -> Compare/2

== system gm_sampleModel2003_1_sub/Subsystem/cfblk7/Positive ==
  u : Inport  OutDataTypeStr=uint8  SampleTime=1
  Compare : RelationalOperator  Operator=>  OutDataTypeStr=boolean  ZeroCross=off
  Constant : Constant  DisableCoverage=on  Value=0  OutDataTypeStr=Inherit: Inherit via back propagation  SampleTime=-1  PreserveConstantTs=on
  y : Outport  SampleTime=1
  wires:
  u/1 -> Compare/1
  Compare/1 -> y/1
  Constant/1 -> Compare/2
